simulink model "SimulationContinueMCC"  (R2017b)
settings: Solver=VariableStepAuto  StartTime=0.0  StopTime=Tf  MaxStep=1e-4  RelTol=1e-3
values from neighbouring files (symbols this model uses):
  C0 = 0.0    (= 0)    [DCMotorParameters.m]    (also in DonneesMCC.m)
  Cl = .0    (= 0)    [DCMotorParameters.m]    (also in DonneesMCC.m)
  F = 0.0001    [DCMotorParameters.m]    (also in DonneesMCC.m)
  J = 2.20e-4    (= 0.00022)    [DCMotorParameters.m]    (also in DonneesMCC.m)
  Kelec = place(Ae,Be,Elec_desired_poles)    [DCMotorParameters.m]    (also in DonneesMCC.m = -place(Ae,Be,Pole_elec_desiree))
  Kmeca = place(Am,Bm,Pole_meca_desiree)    [DCMotorParameters.m]    (also in DonneesMCC.m)
  Kphi = 0.061    [DCMotorParameters.m]    (also in DonneesMCC.m)
  L = 2.7e-3    (= 0.0027)    [DCMotorParameters.m]    (also in DonneesMCC.m)
  R = 1.22    [DCMotorParameters.m]    (also in DonneesMCC.m)
  Ts = 1e-4    (= 0.0001)    [DCMotorParameters.m]    (also in DonneesMCC.m)
settings Model: Creator=romaindelpoux  LastModifiedBy=rdelpoux
settings SolverCC: ZeroCrossControl=DisableAll

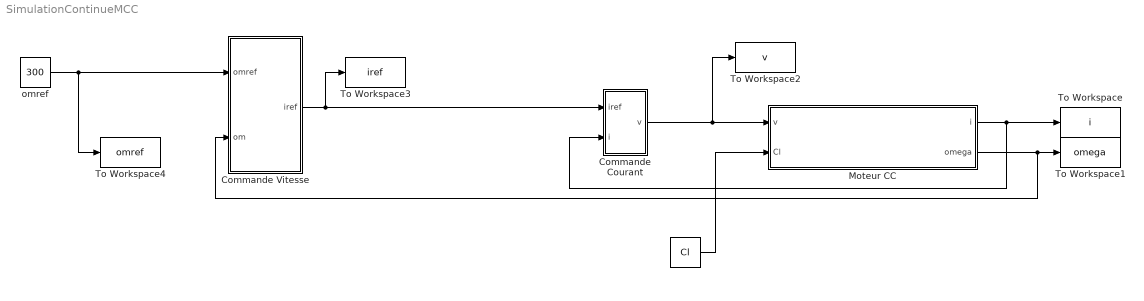
== system SimulationContinueMCC ==
  " " : Constant  Value=Cl
  Commande Courant : Subsystem
  Commande Vitesse : Subsystem
  Moteur CC : Subsystem
  To Workspace : ToWorkspace  VariableName=i  SaveFormat=Timeseries  SampleTime=-1
  To Workspace1 : ToWorkspace  VariableName=omega  SaveFormat=Timeseries  SampleTime=-1
  To Workspace2 : ToWorkspace  VariableName=v  SaveFormat=Timeseries  SampleTime=-1
  To Workspace3 : ToWorkspace  VariableName=iref  SaveFormat=Timeseries  SampleTime=-1
  To Workspace4 : ToWorkspace  VariableName=omref  SaveFormat=Timeseries  SampleTime=-1
  omref : Constant  Value=300
  wires:
  Commande Courant/1(v) -> To Workspace2/1, Moteur CC/1(v)
  Moteur CC/2(omega) -> Commande Vitesse/2(om), To Workspace1/1
  Moteur CC/1(i) -> Commande Courant/2(i), To Workspace/1
  omref/1 -> To Workspace4/1, Commande Vitesse/1(omref)
  Commande Vitesse/1(iref) -> To Workspace3/1, Commande Courant/1(iref)
  " "/1 -> Moteur CC/2(Cl)

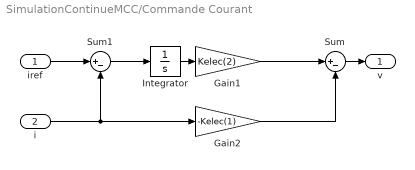
== system SimulationContinueMCC/Commande Courant ==
  iref : Inport
  i : Inport  Port=2
  Gain1 : Gain  Gain=Kelec(2)
  Gain2 : Gain  Gain=-Kelec(1)
  Integrator : Integrator
  Sum : Sum  Inputs=|+-
  Sum1 : Sum  Inputs=|+-
  v : Outport
  wires:
  iref/1 -> Sum1/1
  i/1 -> Gain2/1, Sum1/2
  Integrator/1 -> Gain1/1
  Gain1/1 -> Sum/1
  Sum1/1 -> Integrator/1
  Sum/1 -> v/1
  Gain2/1 -> Sum/2

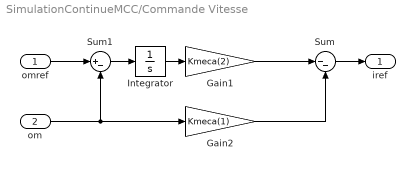
== system SimulationContinueMCC/Commande Vitesse ==
  omref : Inport
  om : Inport  Port=2
  Gain1 : Gain  Gain=Kmeca(2)
  Gain2 : Gain  Gain=Kmeca(1)
  Integrator : Integrator
  Sum : Sum  Inputs=|--
  Sum1 : Sum  Inputs=|+-
  iref : Outport
  wires:
  Gain1/1 -> Sum/1
  Integrator/1 -> Gain1/1
  Sum1/1 -> Integrator/1
  omref/1 -> Sum1/1
  Gain2/1 -> Sum/2
  Sum/1 -> iref/1
  om/1 -> Gain2/1, Sum1/2

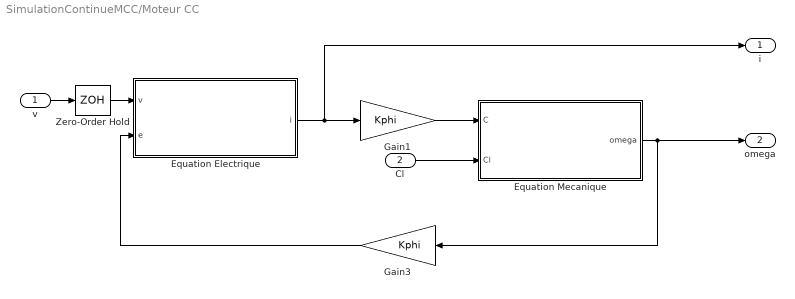
== system SimulationContinueMCC/Moteur CC ==
  v : Inport
  Cl : Inport  Port=2
  Equation Electrique : Subsystem
  Equation Mecanique : Subsystem
  Gain1 : Gain  Gain=Kphi
  "Gain3  " : Gain  Gain=Kphi
  Zero-Order Hold : ZeroOrderHold  SampleTime=Ts
  i : Outport
  omega : Outport  Port=2
  wires:
  v/1 -> Zero-Order Hold/1
  "Gain3  "/1 -> Equation Electrique/2(e)
  Gain1/1 -> Equation Mecanique/1(C)
  Cl/1 -> Equation Mecanique/2(Cl)
  Zero-Order Hold/1 -> Equation Electrique/1(v)
  Equation Electrique/1(i) -> i/1, Gain1/1
  Equation Mecanique/1(omega) -> omega/1, "Gain3  "/1

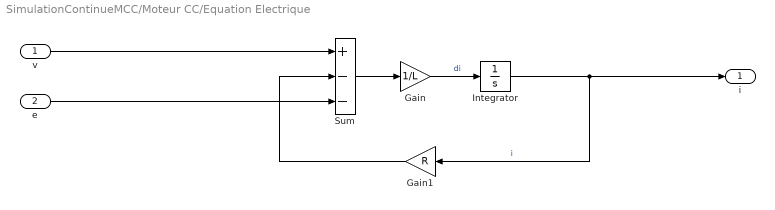
== system SimulationContinueMCC/Moteur CC/Equation Electrique ==
  v : Inport
  e : Inport  Port=2
  Gain : Gain  Gain=1/L
  Gain1 : Gain  Gain=R
  Integrator : Integrator
  Sum : Sum  Inputs=+--
  i : Outport
  wires:
  Gain1/1 -> Sum/2
  Sum/1 -> Gain/1
  Integrator/1 -> i/1, Gain1/1  "i"
  Gain/1 -> Integrator/1  "di"
  v/1 -> Sum/1
  e/1 -> Sum/3

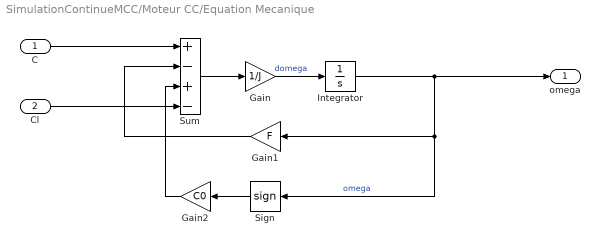
== system SimulationContinueMCC/Moteur CC/Equation Mecanique ==
  C : Inport
  Cl : Inport  Port=2
  Gain : Gain  Gain=1/J
  Gain1 : Gain  Gain=F
  Gain2 : Gain  Gain=C0
  Integrator : Integrator
  Sign : Signum
  Sum : Sum  Inputs=+-+-
  omega : Outport
  wires:
  Gain/1 -> Integrator/1  "domega"
  Integrator/1 -> Sign/1, Gain1/1, omega/1  "omega"
  Sum/1 -> Gain/1
  Gain1/1 -> Sum/2
  Sign/1 -> Gain2/1
  Gain2/1 -> Sum/3
  C/1 -> Sum/1
  Cl/1 -> Sum/4
